simulink model "Vehicle_Hauling"  (Simulink 8.8)
settings: Solver=ode45  StartTime=0  StopTime=85  RelTol=1e-3  EnableMultiTasking=on
libraries: Solver_SF x2
settings Model: Creator=dhall  LastModifiedBy=mkhan  ExtModeTrigMode=oneshot  ExtModeArmWhenConnect=off
settings DataIOCC: LimitDataPoints=off  SignalLoggingName=sigsOut
settings OptimizationCC: BooleanDataType=off  LocalBlockOutputs=off  InitFltsAndDblsToZero=on
settings DebuggingCC: SaveWithParameterizedLinksMsg=none  SignalResolutionControl=TryResolveAllWithWarning  MultiTaskDSMMsg=warning  MultiTaskCondExecSysMsg=none  SFExecutionAtInitializationDiag=warning
settings HardwareCC: TargetUnknown=on
settings GRTTargetCC: TargetFcnLib=ansi_tfl_tmw.mat  CompOptLevelCompliant=off
settings ConfigComp: CovSFcnEnable=off

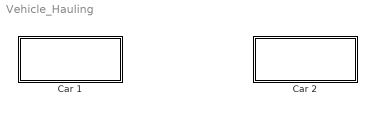
== system Vehicle_Hauling ==
  Car 1 : Subsystem
  Car 2 : Subsystem

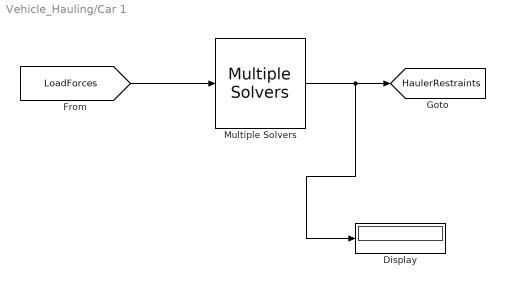
== system Vehicle_Hauling/Car 1 ==
  Display : Display
  Multiple Solvers : Solver_SF/Multiple Solvers  Priority=1  iVehicle=1  SIMFILE=D:\product_dev\trunk\Image\CarSim\Core\CarSim_Data\Extensions\Simulink\Parallel_Solver\simfile1.sim  Run_RTs=off  vs_state_ind=Run  StopMode_ind=Vehicle Model  vs_scx=on
  tag scope: HaulerRestraints=global
  wires:
  Multiple Solvers/1 -> Display/1, [HaulerRestraints]
  [LoadForces] -> Multiple Solvers/1

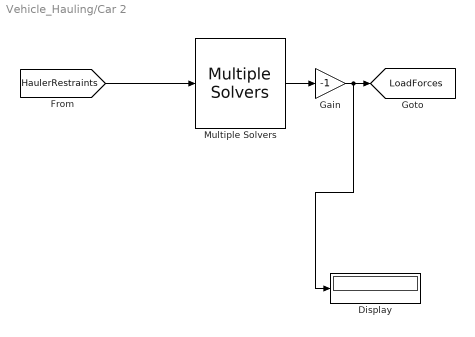
== system Vehicle_Hauling/Car 2 ==
  Display : Display
  Gain : Gain  Gain=-1
  Multiple Solvers : Solver_SF/Multiple Solvers  Priority=1  iVehicle=2  SIMFILE=D:\product_dev\trunk\Image\CarSim\Core\CarSim_Data\Extensions\Simulink\Parallel_Solver\simfile2.sim  Run_RTs=off  vs_state_ind=Run  StopMode_ind=Vehicle Model  vs_scx=on
  tag scope: LoadForces=global
  wires:
  Multiple Solvers/1 -> Gain/1
  [HaulerRestraints] -> Multiple Solvers/1
  Gain/1 -> Display/1, [LoadForces]
